simulink model "AberrantEyes6"  (R2014b)
settings: Solver=ode45  StartTime=0.0  StopTime=inf  FixedStep=1/120  RelTol=1e-3
StopFcn:
  | format shortg
  | c = clock;
  | log_filename = ['log_ETT_',num2str(c(1)),'_',num2str(c(2)),'_',num2str(c(3)),'_',num2str(c(4)),'_',num2str(c(5)),'_',num2str(round(c(6)))];
  | save(log_filename,'eyeres')
libraries: simulink x3, dspswit3 x2, dspnetwork x2, RT x1
settings Model: Creator=SmartEye DR120  LastModifiedBy=SmartEye DR120
settings DataIOCC: LimitDataPoints=off  SaveOutput=off  SignalLogging=off  DSMLogging=off  VisualizeSimOutput=off  SaveTime=off

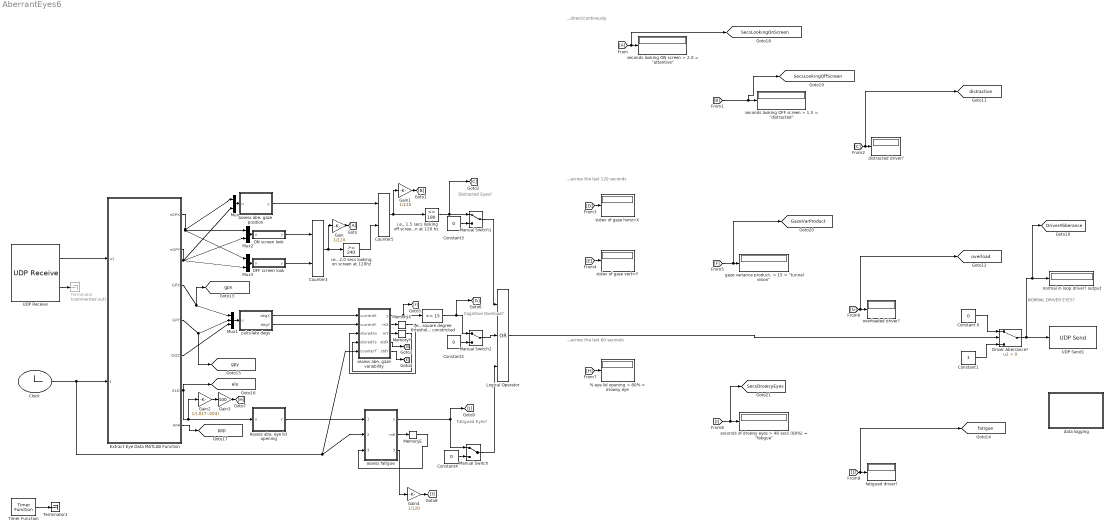
== system AberrantEyes6 ==
  note: Distracted
      | Eyes?
  note: Fatigued
      | Eyes?
  note: NORMAL DRIVER EYES?
  note: Cognitive
      | Overload?
  note: ...direct/continously
  note: ...across the last 120 seconds
  note: ...across the last 60 seconds
  " gaze variance product, < 15 = \"tunnel vision\"" : Display
  " seconds of drowsy eyes > 48 secs (80%) = \"fatigue\"" : Display
  "% eye lid opening < 80% = drowsy eye " : Display
  Assess abe. eye lid opening : MATLAB Function  TreatAsAtomicUnit=on
  Assess abe. gaze position : MATLAB Function  TreatAsAtomicUnit=on
  Clock : Clock
  Constant 0 : Constant  Value=0
  Constant1 : Constant
  Constant2 : Constant  Value=0
  Constant3 : Constant  Value=0
  Constant4 : Constant  Value=0
  Counter3 : dspswit3/Counter  Direction=Up  CountEvent=Non-zero sample  CounterSize=16 bits  MaxCount=3600  InitialCount=0  Output=Count  HitValue=32  ResetInput=on  SamplesPerFrame=1  Ts=1  CntDtype=uint16  HitDtype=Logical
  Counter5 : dspswit3/Counter  Direction=Up  CountEvent=Non-zero sample  CounterSize=16 bits  MaxCount=3600  InitialCount=0  Output=Count  HitValue=32  ResetInput=on  SamplesPerFrame=1  Ts=1  CntDtype=uint16  HitDtype=Logical
  "Driver Aberrance? " : Switch  Criteria=u2 > Threshold
  Extract Eye Data MATLAB Function : MATLAB Function  TreatAsAtomicUnit=on
  Gain : Gain  Gain=1/120
  Gain1 : Gain  Gain=1/120
  Gain2 : Gain  Gain=1/(.017-.004)
  Gain3 : Gain  Gain=100
  Gain4 : Gain  Gain=1/120
  Logical Operator : Logic  Operator=OR  Inputs=3  AllPortsSameDT=off  OutDataTypeStr=boolean
  Manual Switch : ManualSwitch
  Manual Switch1 : ManualSwitch
  Manual Switch2 : ManualSwitch
  MemoryE : Memory  X0=zeros(1,7200)
  MemoryX : Memory  X0=zeros(1,14400)
  MemoryY : Memory  X0=zeros(1,14400)
  Mux : Mux  Inputs=2
  Mux1 : Mux  Inputs=3
  Mux2 : Mux  Inputs=2
  Mux3 : Mux  Inputs=2
  OFF screen look : MATLAB Function  TreatAsAtomicUnit=on
  ON screen look : MATLAB Function  TreatAsAtomicUnit=on
  Terminator : Terminator  Commented=on
  Terminator1 : Terminator
  Timer Function : RT/Timer Function  step=16.666666  priority=HIGH  ThPriority=TIME CRITICAL
  UDP Receive : dspnetwork/UDP Receive  localURL='0.0.0.0'  localPort=139  remoteURL='192.168.101.1'  remotePort=-1  recvBufferSize=100  dims=100  signalDatatype=uint8  isVarSize=off  showBlockingTime=off  blockingTime=0  sampletime=1/60
  UDP Send1 : dspnetwork/UDP Send  remoteURL='169.254.71.50'  remotePort=25000  localURL='0.0.0.0'  localPortSource=Automatically determine  localPort=-1  sampletime=-1  separateLengthPort=0
  assess abe. gaze variability : MATLAB Function  TreatAsAtomicUnit=on
  assess fatigue : MATLAB Function  TreatAsAtomicUnit=on
  "calculate degs " : MATLAB Function  TreatAsAtomicUnit=on
  data logging : Subsystem
  distracted driver? : Display
  fatigued driver? : Display
  "i.e., square degree threshold for being constricted" : simulink/Logic and Bit Operations/Compare To Constant  relop=<=  const=15  OutDataTypeStr=boolean
  "i.e., 1.5 secs looking off screen at 120 hz" : simulink/Logic and Bit Operations/Compare To Constant  relop=>=  const=180  OutDataTypeStr=boolean
  "i.e., 2.0 secs looking on screen at 120hz" : simulink/Logic and Bit Operations/Compare To Constant  relop=>=  const=240  OutDataTypeStr=boolean
  "normal in loop driver? output " : Display
  overloaded driver? : Display
  "seconds looking OFF screen > 1.5 = \"distracted\"" : Display
  "seconds looking ON screen > 2.0 = \"attentive\"" : Display
  stdev of gaze horiz=X : Display
  stdev of gaze vert=Y : Display
  tag scope: DriverAbberance=global, GazeVarProduct=global, SecsDrowsyEyes=global, SecsLookingOffScreen=global, SecsLookingOnScreen=global, distraction=global, elo=global, fatigue=global, gpx=global, gpy=global, overload=global, ppp=global
  wires:
  UDP Receive/2 -> Terminator/1
  Logical Operator/1 -> "Driver Aberrance? "/2
  Mux/1 -> Assess abe. gaze position/1(u)
  Mux1/1 -> "calculate degs "/1(u)
  Extract Eye Data MATLAB Function/6(ELO) -> Assess abe. eye lid opening/1(u), Gain2/1, [elo]
  "Driver Aberrance? "/1 -> UDP Send1/1, [DriverAbberance], "normal in loop driver? output "/1
  UDP Receive/1 -> Extract Eye Data MATLAB Function/1(u1)
  Timer Function/1 -> Terminator1/1
  Clock/1 -> Extract Eye Data MATLAB Function/2(t), assess fatigue/2(counterT), assess abe. gaze variability/5(counterT)
  Assess abe. eye lid opening/1(y) -> assess fatigue/1(currentE)
  Constant2/1 -> Manual Switch2/2
  Constant3/1 -> Manual Switch1/2
  Constant4/1 -> Manual Switch/2
  Manual Switch/1 -> Logical Operator/3
  Manual Switch2/1 -> Logical Operator/2
  Manual Switch1/1 -> Logical Operator/1
  Counter5/1 -> "i.e., 1.5 secs looking off screen at 120 hz"/1, Gain1/1
  Mux2/1 -> ON screen look/1(u)
  Assess abe. gaze position/1(y) -> Counter5/1
  "i.e., 1.5 secs looking off screen at 120 hz"/1 -> [C], Manual Switch1/1
  Extract Eye Data MATLAB Function/1(nGPX) -> Mux3/1, Mux2/1, Mux/1
  Extract Eye Data MATLAB Function/2(nGPY) -> Mux2/2, Mux3/2, Mux/2
  "i.e., 2.0 secs looking on screen at 120hz"/1 -> Counter5/2
  ON screen look/1(y) -> Counter3/1
  OFF screen look/1(y) -> Counter3/2
  Mux3/1 -> OFF screen look/1(u)
  Extract Eye Data MATLAB Function/5(GOZ) -> Mux1/3
  assess abe. gaze variability/2(mX) -> MemoryX/1
  assess abe. gaze variability/3(mY) -> MemoryY/1
  "calculate degs "/1(degX) -> assess abe. gaze variability/1(currentX)
  "calculate degs "/2(degY) -> assess abe. gaze variability/2(currentY)
  MemoryY/1 -> assess abe. gaze variability/4(storedYs)
  MemoryX/1 -> assess abe. gaze variability/3(storedXs)
  assess abe. gaze variability/1(y) -> [F], "i.e., square degree threshold for being constricted"/1
  Extract Eye Data MATLAB Function/4(GPY) -> [gpy], Mux1/2
  Extract Eye Data MATLAB Function/3(GPX) -> [gpx], Mux1/1
  assess fatigue/2(mE) -> MemoryE/1
  MemoryE/1 -> assess fatigue/3(storedEs)
  Constant1/1 -> "Driver Aberrance? "/3
  Constant 0/1 -> "Driver Aberrance? "/1
  "i.e., square degree threshold for being constricted"/1 -> [G], Manual Switch2/1
  Counter3/1 -> "i.e., 2.0 secs looking on screen at 120hz"/1, Gain/1
  Gain2/1 -> Gain3/1
  assess fatigue/3(badEyeOpenings) -> Gain4/1
  Gain/1 -> [A]
  [A] -> [SecsLookingOnScreen], "seconds looking ON screen > 2.0 = \"attentive\""/1
  Gain1/1 -> [B]
  assess abe. gaze variability/4(stdX) -> [D]
  [D] -> stdev of gaze horiz=X/1
  assess abe. gaze variability/5(stdY) -> [E]
  [E] -> stdev of gaze vert=Y/1
  [F] -> [GazeVarProduct], " gaze variance product, < 15 = \"tunnel vision\""/1
  [G] -> [overload], overloaded driver?/1
  Gain3/1 -> [H]
  [H] -> "% eye lid opening < 80% = drowsy eye "/1
  Gain4/1 -> [I]
  [I] -> [SecsDrowsyEyes], " seconds of drowsy eyes > 48 secs (80%) = \"fatigue\""/1
  assess fatigue/1(y) -> [J], Manual Switch/1
  [J] -> [fatigue], fatigued driver?/1
  [C] -> [distraction], distracted driver?/1
  Extract Eye Data MATLAB Function/7(PPP) -> [ppp]
  [B] -> [SecsLookingOffScreen], "seconds looking OFF screen > 1.5 = \"distracted\""/1

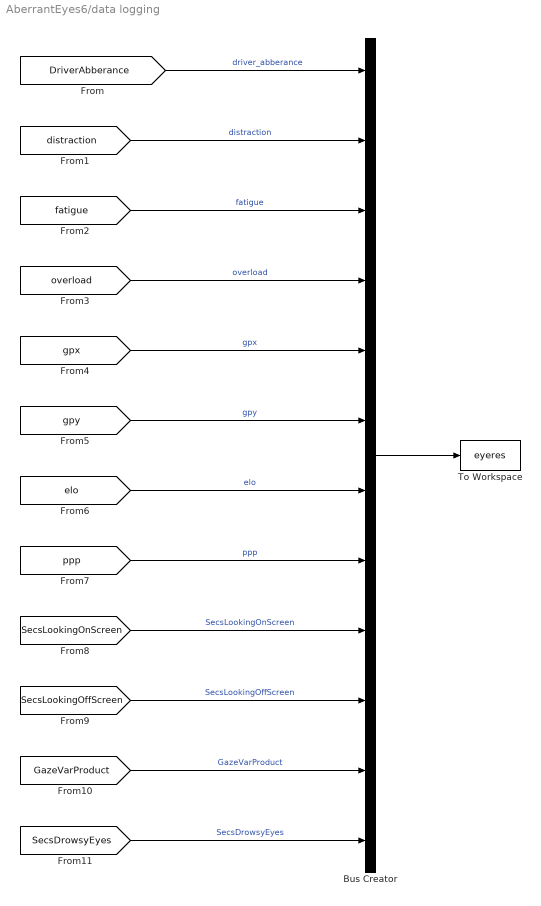
== system AberrantEyes6/data logging ==
  Bus Creator : BusCreator  Inputs='driver_abberance','distraction','fatigue','overload','gpx','gpy','elo','ppp','SecsLookingOnScreen','SecsLookingOffScreen','GazeVarProduct','SecsDrowsyEyes'
  To Workspace : ToWorkspace  VariableName=eyeres  SaveFormat=Timeseries  SampleTime=-1
  wires:
  Bus Creator/1 -> To Workspace/1
  [DriverAbberance] -> Bus Creator/1  "driver_abberance"
  [distraction] -> Bus Creator/2  "distraction"
  [fatigue] -> Bus Creator/3  "fatigue"
  [overload] -> Bus Creator/4  "overload"
  [gpx] -> Bus Creator/5  "gpx"
  [gpy] -> Bus Creator/6  "gpy"
  [elo] -> Bus Creator/7  "elo"
  [ppp] -> Bus Creator/8  "ppp"
  [SecsLookingOnScreen] -> Bus Creator/9  "SecsLookingOnScreen"
  [SecsLookingOffScreen] -> Bus Creator/10  "SecsLookingOffScreen"
  [GazeVarProduct] -> Bus Creator/11  "GazeVarProduct"
  [SecsDrowsyEyes] -> Bus Creator/12  "SecsDrowsyEyes"

== matlab function AberrantEyes6/Extract Eye Data MATLAB Function ==
  settings: sampleTime=1/120
  data: u1 input; t input; nGPX output; nGPY output; GPX output; GPY output; GOZ output; ELO output; PPP output
function [nGPX,nGPY,GPX,GPY,GOZ,ELO,PPP] = fcn(u1,t)
%#codegen
if t == 0
    u1 = uint8(zeros(100,1));
end

%initial layer
X = 0;
Y = 0;
Z = 0;
Q = 0;
OX = 0;
OY = 0;
OZ = 0;
EO = 0;
PP = 0;

%intermediate layer
GDX = 0;
GDY = 0;
GDZ = 0;
GOX = 0;
GOY = 0;
GOZ = 0;
GDQ = 0;
ELO = 0;
PPP = 0;

%second intermediate layer
GPX = 0;
GPY = 0;


%final layer
nGPX = 0;
nGPY = 0;

%access addresses of data separate from headers and from each other in
%various subpackets of the UDP full packet message
OX(1) = typecast(uint8(u1(13:20)),'double');
OY(1) = typecast(uint8(u1(21:28)),'double');
OZ(1) = typecast(uint8(u1(29:36)),'double');
X(1) = typecast(uint8(u1(41:48)),'double');
Y(1) = typecast(uint8(u1(49:56)),'double');
Z(1) = typecast(uint8(u1(57:64)),'double');
Q(1) = typecast(uint8(u1(69:76)),'double');
EO(1) = typecast(uint8(u1(81:88)),'double');
PP(1) = typecast(uint8(u1(93:100)),'double');

%assign to intermediate layer
GOX(1) = swapbytes(OX(1));
GOY(1) = swapbytes(OY(1));
GOZ(1) = swapbytes(OZ(1));
GDX(1) = swapbytes(X(1));
GDY(1) = swapbytes(Y(1));
GDZ(1) = swapbytes(Z(1));
GDQ(1) = swapbytes(Q(1));
ELO(1) = swapbytes(EO(1));
PPP(1) = swapbytes(PP(1));



%% Calculate Gaze Point that falls on the plane above the cameras
% based on gaze origin distance info and gaze direction angles
M_yz = sqrt(GDY^2+GDZ^2);
M_xz = sqrt(GDX^2+GDZ^2);
if M_yz == 0 && M_xz == 0
    M_yz = 0.01;
    M_xz = 0.01;
end
Theta_MZ_X = acos(abs(GDZ/M_xz));
Theta_MZ_Y = acos(abs(GDZ/M_yz));

GPX = GOX + sign(GDX)*GOZ*tan(Theta_MZ_X);
GPY = GOY + sign(GDY)*GOZ*tan(Theta_MZ_Y);


%% Define Monitor Surface Gaze Point upper and lower bounds relative to "center" camera location
GPBX_LOW = -0.26; %left screen edge boundary, meters
GPBX_UP = 0.26; %right screen edge boundary, meters

GPBY_LOW = 0.055; %lower screen edge boundary, meters
GPBY_UP = 0.385; %upper screen edge boundary, meters



%%Normalize Gaze Point around a 0,0 (x,y) in center of screen such that 
% x positive = right, x negative = left
% y positive = top, y negative = bottom
%(x,y)
% 1,1 = top right corner
% 1,-1 = bottom right corner
% -1,-1 = bottom left corner
% -1,1 = top left corner

%take steps to normalize gaze position data
%offset = abs(0 - min)
%newMid = ((min - offset) + (max - offset))/2
%%out = -1 * ((in - offset) - newMid)*(1/newMid); full range spans 0
%%out = ((in - offset) - newMid)*(1/newMid) full range is above 0

offsetX = abs(0 - GPBX_LOW);
newMidX = ((GPBX_LOW-offsetX)+(GPBX_UP-offsetX))/2;
nGPX = -1 * ((GPX - offsetX) - newMidX)*(1/newMidX);

offsetY = abs(0 - GPBY_LOW);
newMidY = ((GPBY_LOW-offsetY)+(GPBY_UP-offsetY))/2;
nGPY =  ((GPY - offsetY) - newMidY)*(1/newMidY);

== matlab function AberrantEyes6/Assess abe. gaze position ==
  data: u input; y output
function y = fcn(u)
%#codegen

nGPX = u(1);
nGPY = u(2);

abeGazeLoc = 0;

if (or(or(nGPX>1,nGPX<-1),or(nGPY>1,nGPY<-1)))||(nGPX==0&&nGPY==0)
    abeGazeLoc = 1;
else
    abeGazeLoc = 0; 
end

y = abeGazeLoc;

== matlab function AberrantEyes6/Assess abe. eye lid opening ==
  data: u input; y output
function y  = fcn(u)
%#codegen

%current eyelid opening value
ELO = u(1);

%initial default assessment of current eyelid opening value 
abeELO =  0;

%default measured, a priori min/max values of ELO
fullOpen = 0.017;
fullClosed = 0.004;

%trigger if less than threshold... ... ...
%trigger less often
%conTrigThresh = fullClosed + (0.20 * (fullOpen - fullClosed));
%trigger more often
libTrigThresh = fullClosed + (0.80 * (fullOpen - fullClosed));

%current assessment of ELO as aberrant or not
if ELO < libTrigThresh
    %score a current "bad" value
    abeELO =  1;
else
    %score a current "ok" value
    abeELO =  0;
end

y = abeELO;


%{


if t>0
    %first pass through ... fill up 1 minute of values
    %add current abeELO assessment to storage space
    if t < 60
        %just fill sequentially forwards
        timeWindow(t(1/60)) = abeELO;
        
        %provide default ok state for fatigue
        y = 0;
    end
    
    %after one full minute and forever onwards...
    if t >= 60
        %first shift, moves last value over to second to last position
        timeWindow((length(timeWindow)-1)) = timeWindow(length(timeWindow));
    
        %last position in timeWindow gets the current ELO assessment value
        timeWindow(length(timeWindow)) = abeELO;
    
        %assess FATIGUE state 1 or 0
        %assess aross the (minute) time window, # of trigger values
        %trigger Fatigue state if 80% or more of (minute) time window is "bad"
        if sum(timeWindow==1) >= (.80*length(timeWindow))
            y = 1;
        else
            y = 0;
        end
        
        %shift all the other values/positions over, excepting the last two
        for i = 1:(length(timeWindow)-2)
            timeWindow(i)= timeWindow(i+1);
        end
    
else
    %provide default ok state for fatigue
    y = 0;
end


%%%%in the first step of full model
%create a window of time equal to  ...
%3600 is a full minute of samples, at 60 samples a second
%if t == 0
  % assignin('base','tmeWindow',zeros(1,3600));
%end


%initialize a timeWindow storage space somwhere...
%model workspace?? ...'base' matlab base worksapce??
%timeWindow = (zeros(1,3600))

%}

== matlab function AberrantEyes6/calculate degs  ==
  data: u input; degX output; degY output
function [degX,degY] = fcn(u)
%#codegen

GPX = u(1);
GPY = u(2);
GOZ = u(3);

%calculate degrees in X and Y from 0,0 origin in middle of screen
degX = (180/pi)*(atan(GPX/GOZ));
degY = (180/pi)*(atan(GPY/GOZ));

== matlab function AberrantEyes6/OFF screen look ==
  data: u input; y output
function y = fcn(u)
%#codegen

nGPX = u(1);
nGPY = u(2);

offScreen = 0;

if nGPX > 1 || nGPX < -1 || nGPY > 1 || nGPY < -1.334
    offScreen = 1;
else
    offScreen = 0;
end


y = offScreen;

== matlab function AberrantEyes6/ON screen look ==
  data: u input; y output
function y = fcn(u)
%#codegen

nGPX = u(1);
nGPY = u(2);

onScreen = 0;

%if (or(and(nGPX<=1,nGPX>=-1),and(nGPY<=1,nGPY>=-1)))&&(nGPX~=0)&&(nGPY~=0)
%    reset = 1;
%else
%    reset = 0; 
%end

if nGPX<=1&&nGPX>=-1&&nGPX~=0&&nGPY<=1&&nGPY>=-1&&nGPY~=0
    onScreen = 1;
else
    onScreen = 0;
end

%if nGPY<=1&&nGPY>=-1
%    reset = 1;
%end


y = onScreen;

== matlab function AberrantEyes6/assess fatigue ==
  data: currentE input; counterT input; storedEs input; y output; mE output; badEyeOpenings output
function [y,mE,badEyeOpenings] = fcn(currentE,counterT,storedEs)
%#codegen

%3600 is 60 seconds at 60 per second 
%7200 is 60 seconds at 120 per second 
%also set in MemoryE

newStoreE = zeros(1,7200);
mE = zeros(1,7200);
fatigue = 0;

newStoreE(1:7199) = storedEs(2:end);
if isnan(currentE)%block nan values
    newStoreE(7200) = storedEs(422);%sample from storage pseudo randomly
else
    newStoreE(7200) = currentE;
end

mE = newStoreE;

%1 minutes  = 60 secs
if counterT > 60
    if sum(newStoreE == 1) >= 5760 %80 percent of 1 minute of samples at 120hz
        fatigue = 1;
    end
else
    fatigue = 0; 
end

badEyeOpenings = sum(newStoreE == 1);

y = fatigue;

== matlab function AberrantEyes6/assess abe. gaze variability ==
  data: currentX input; currentY input; storedXs input; storedYs input; y output; mX output; counterT input; mY output; stdX output; stdY output
function [y,mX,mY,stdX,stdY] = fcn(currentX,currentY,storedXs,storedYs,counterT)
%#codegen

%600 is ten seconds at 60 per second 
%7200 is 2 minutes at 60 per second
%14400 is 2 minutes at 120 per second
%also set in MemoryX and MemoryY obj blocks intial condition field
sqDegGazeVar = 630.0;%approx max value of covering whole screen
newStoreX = zeros(1,14400);
newStoreY = zeros(1,14400);
mX = zeros(1,14400);
mY = zeros(1,14400);

newStoreX(1:14399) = storedXs(2:end);
if isnan(currentX)%block nan values
    newStoreX(14400) = storedXs(717);%sample from storage pseudo randomly
else
    newStoreX(14400) = currentX;
end

newStoreY(1:14399) = storedYs(2:end);
if isnan(currentY)%block nan values
    newStoreY(14400) = storedYs(422);%sample from storage pseudo randomly
else
    newStoreY(14400) = currentY;
end

mX = newStoreX;
mY = newStoreY;

%2 minutes seconds = 120 secs
if counterT > 120
    %compute a square degree gaze variance product of standard deviations
    sqDegGazeVar = std(newStoreX) * std(newStoreY);
else
    sqDegGazeVar = 630.0; %max screen covereage (-21:21 degs x; 5:35 degs y)
end

stdX = std(newStoreX);
stdY = std(newStoreY);

y = sqDegGazeVar;
